simulink subsystem "SystemInputsSimMotorSwap"  (R2024b)
settings: Solver=VariableStepAuto  StartTime=0.0  StopTime=10.0  RelTol=1e-3
values from neighbouring files (symbols this model uses):
  Ts = T_pwm    [mcbMotorSwapData.m]
undefined symbols (not defined in the file or in its folder): pmsm
libraries: simulink x1, mcbpmsmparamestlib x1
settings Model: Creator=The MathWorks, Inc.  LastModifiedBy=snarayan
settings RTWCC: GPUComputeCapability=3.5

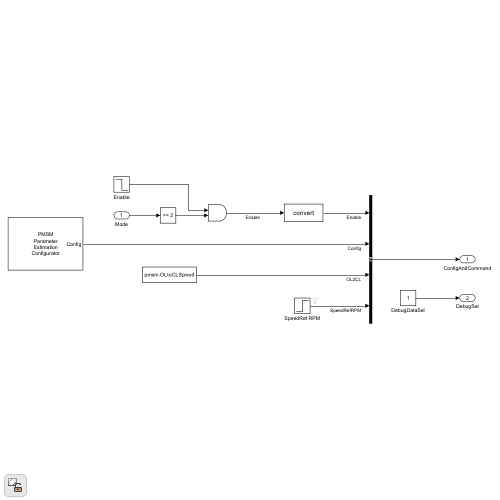
[thumbnail: Simulink's stored preview of the top-level diagram]
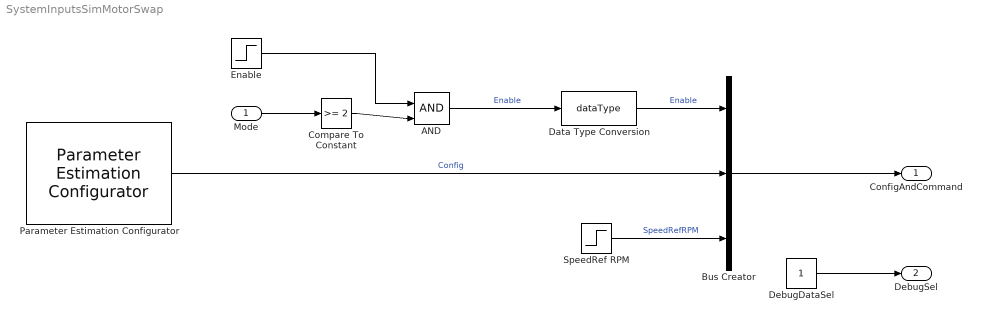
== system SystemInputsSimMotorSwap ==
  Mode : Inport
  AND : Logic  IconShape=distinctive  AllPortsSameDT=off  OutDataTypeStr=boolean
  Bus Creator : BusCreator  Inputs=3
  Compare To Constant : simulink/Logic and Bit Operations/Compare To Constant  relop=>=  const=2  OutDataTypeStr=boolean
  Data Type Conversion : DataTypeConversion  OutDataTypeStr=dataType  RndMeth=Simplest  SaturateOnIntegerOverflow=off
  DebugDataSel : Constant  OutDataTypeStr=uint8  SampleTime=-1
  Enable : Step  Time=100  Before=1  After=0  OutDataTypeStr=dataType
  Parameter Estimation Configurator : mcbpmsmparamestlib/Parameter Estimation Configurator  P=pmsm.p  NRated=pmsm.N_rated  IRated=pmsm.I_rated  ImaxInverter=inverter.ISenseMax  RBoard=inverter.R_board  ISenseGain=inverter.AMPPerCount  VSenseGain=inverter.VoltPerCount  FreqMax=1000  FreqMin=400  FreqStepSweep=100  FreqStepEst=10  FreqNum=10  CurrMeasDelay=2*Ts  KeTime=3  KeSpeed=pmsm.N_rated * 0.8  IqRefFOC=0.2  KpKiInputEnable=off  Kp=1  Ki=1000  JSpeedLow=pmsm.N_rated * 0.3  DataType=single  Ts=Ts
      settings: LibrarySourceBlock=mcblib/Parameter Estimation/PMSM Parameter Estimation/Parameter Estimation Configurator
  SpeedRef RPM : Step  Time=28  Before=pmsm.N_rated * 0.5  After=pmsm.N_rated * 0.8  OutDataTypeStr=dataType
  ConfigAndCommand : Outport
  DebugSel : Outport  Port=2
  wires:
  DebugDataSel/1 -> DebugSel/1
  SpeedRef RPM/1 -> Bus Creator/3  "SpeedRefRPM"
  Enable/1 -> AND/1
  Data Type Conversion/1 -> Bus Creator/1  "Enable"
  Mode/1 -> Compare To Constant/1
  Bus Creator/1 -> ConfigAndCommand/1
  Compare To Constant/1 -> AND/2
  Parameter Estimation Configurator/1 -> Bus Creator/2  "Config"
  AND/1 -> Data Type Conversion/1  "Enable"
